simulink model "ModelTesting"  (R2024b)
settings: Solver=VariableStepAuto  StartTime=0.0  StopTime=10.0  RelTol=1e-3
model workspace (MAT data in the model file):
  l = 40
  r = 8
settings Model: Creator=Matthew  LastModifiedBy=Matthew

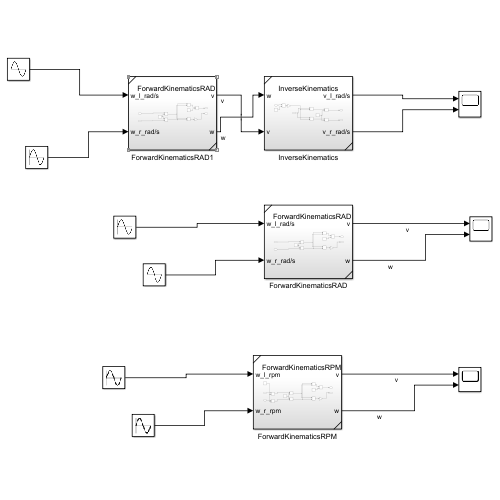
[thumbnail: Simulink's stored preview of the top-level diagram]
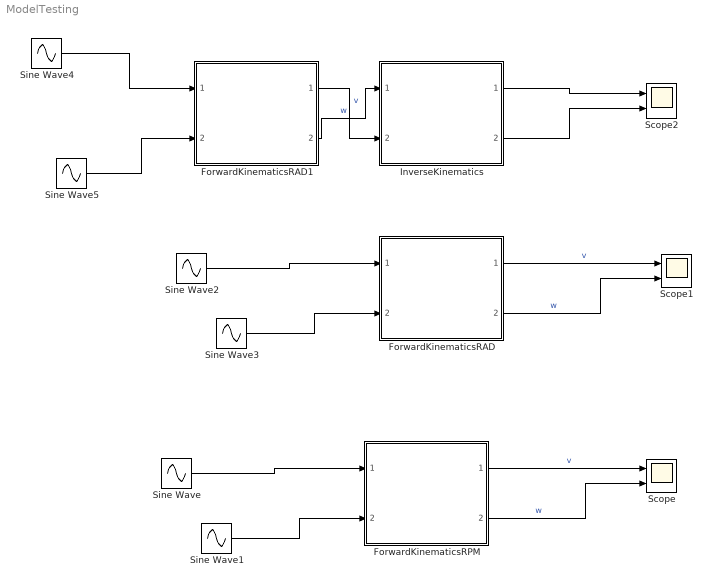
== system ModelTesting ==
  ForwardKinematicsRAD : Subsystem  ReferencedSubsystem=ForwardKinematicsRAD
  ForwardKinematicsRAD1 : Subsystem  ReferencedSubsystem=ForwardKinematicsRAD
  ForwardKinematicsRPM : Subsystem  ReferencedSubsystem=ForwardKinematicsRPM
  InverseKinematics : Subsystem  ReferencedSubsystem=InverseKinematics
  Scope : Scope  NumInputPorts=2
  Scope1 : Scope  NumInputPorts=2
  Scope2 : Scope  NumInputPorts=2
  Sine Wave{,1..5} (6 alike) : Sin  SampleTime=0
  wires:
  ForwardKinematicsRPM/1 -> Scope/1  "v"
  ForwardKinematicsRPM/2 -> Scope/2  "w"
  Sine Wave/1 -> ForwardKinematicsRPM/1
  Sine Wave1/1 -> ForwardKinematicsRPM/2
  Sine Wave3/1 -> ForwardKinematicsRAD/2
  ForwardKinematicsRAD/2 -> Scope1/2  "w"
  ForwardKinematicsRAD/1 -> Scope1/1  "v"
  Sine Wave2/1 -> ForwardKinematicsRAD/1
  Sine Wave4/1 -> ForwardKinematicsRAD1/1
  Sine Wave5/1 -> ForwardKinematicsRAD1/2
  InverseKinematics/1 -> Scope2/1
  InverseKinematics/2 -> Scope2/2
  ForwardKinematicsRAD1/1 -> InverseKinematics/2  "v"
  ForwardKinematicsRAD1/2 -> InverseKinematics/1  "w"
